simulink library "MERMASS11MSEREF"  (R2020b)
settings: Solver=ode45  StartTime=0.0  StopTime=10.0  RelTol=1e-3  EnableMultiTasking=on
settings Model: Creator=vda2sh  LastModifiedBy=CAV2OFO
settings DataIOCC: LimitDataPoints=on  SaveFormat=Array  ReturnWorkspaceOutputs=off
settings OptimizationCC: LifeSpan=inf
settings DebuggingCC: SolverPrmCheckMsg=warning  SFUnexpectedBacktrackingDiag=warning  SFNoUnconditionalDefaultTransitionDiag=warning  SFExecutionAtInitializationDiag=none  ArithmeticOperatorsInVariantConditions=warning
settings HardwareCC: ProdBitPerPointer=32  ProdBitPerSizeT=32  ProdBitPerPtrDiffT=32  ProdLargestAtomicFloat=None  ProdIntDivRoundTo=Undefined  ProdEndianess=Unspecified  ProdWordSize=32  ProdHWDeviceType=32-bit Generic
settings ModelReferenceCC: PropagateSignalLabelsOutOfModel=off
settings SFSimCC: SimUseLocalCustomCode=off  CustomCodeUndefinedFunction=UseInterfaceOnly
settings RTWCC: RTWUseLocalCustomCode=off
settings CodeAppCC: StateflowObjectComments=on
settings GRTTargetCC: TargetLangStandard=C89/C90 (ANSI)
settings ConfigComp: CovMetricSettings=dw  CovSaveCumulativeToWorkspaceVar=on  CovSaveSingleToWorkspaceVar=on  CovExternalEMLEnable=off  CovSFcnEnable=off

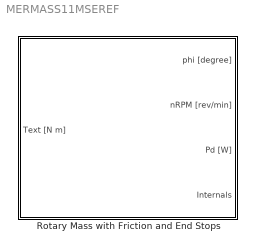
== system MERMASS11MSEREF ==
  Rotary Mass with Friction and End Stops : Subsystem  Tag=MERMASS11MSEREF  mask(MERMASS11MSEREF){J=1.625e-5, dvisc=0.001, frictionmode=no friction, epsn=0.001, tauinv=1000, TStick=1, TCoulomb=0.9, nStri=0.01, endstopmode=no end stop, phimin=-1e6, phimax=1e6, cstop=1e6, kimpact=0.5, phiinit=0, nRPMinit=0}
      mask prompts: J "Inertia [kg m2]"; dvisc "Viscous damping [N m/(rev/min)]"; frictionmode "Friction mode"; epsn "Numerical parameter for friction treatment [rev/min]"; tauinv "Inverse of time constant at stiction (variable step solvers only) [1/s]"; TStick "Torque at stick friction [N m]"; TCoulomb "Torque at Coulomb friction [N m]"; nStri "Stribeck rotational speed [rev/min]"; endstopmode "End stop mode"; phimin "Lower angular displacement limit [°]"; phimax "Upper angular displacement limit [°]"; cstop "Spring coefficient at displacement limit [N m/°]"; kimpact "Coefficient of restitution [-]"; phiinit "Initial displacement [°]"; nRPMinit "Initial rotational speed [rev/min]"
      mask help:
      | MERMASS11MSEREF - Rotary Mass with Friction and End Stops
      |
      | This is a model of a mass in rotary motion with friction effects and inertia. The displacement of the mass may be limited by lower and upper values. One detailed model of friction is implemented, as well as one model for the phenomenon of end stop.
      settings: AttributesFormatString=<%<Tag>>
      mask Help: eval('show_docs_mseref_mechanics(''MERMASS11MSEREF'')')
      mask TypeOptions frictionmode: no friction | stribeck + slip/Coulomb friction
      mask Callback frictionmode:
      | MCBVP__.endstopmode = get_param(gcb,'endstopmode');
      | 
      | MCBVP__.frictionmode = get_param(gcb,'frictionmode');
      | 
      | 		MCBVP__.enables = {};
      | 		MCBVP__.visibilities = {};
      | 
      | 				MCBVP__.enables{end + 1} = 'on';
      | 				MCBVP__.visibilities{end + 1} = 'on';
      | 
      | 				MCBVP__.enables{end + 1} = 'on';
      | 				MCBVP__.visibilities{end + 1} = 'on';
      | 
      | 				MCBVP__.enables{end + 1} = 'on';
      | 				MCBVP__.visibilities{end + 1} = 'on';
      | 
      | 				if strcmp(MCBVP__.frictionmode,'stribeck + slip/Coulomb friction')
      | 					MCBVP__.enables{end + 1} = 'on';
      | 					MCBVP__.visibilities{end + 1} = 'on';
      | 				else
      | 					MCBVP__.enables{end + 1} = 'off';
      | 					MCBVP__.visibilities{end + 1} = 'off';
      | 				end
      | 
      | 				if strcmp(MCBVP__.frictionmode,'stribeck + slip/Coulomb friction')
      | 					MCBVP__.enables{end + 1} = 'on';
      | 					MCBVP__.visibilities{end + 1} = 'on';
      | 				else
      | 					MCBVP__.enables{end + 1} = 'off';
      | 					MCBVP__.visibilities{end + 1} = 'off';
      | 				end
      | 
      | 				if strcmp(MCBVP__.frictionmode,'stribeck + slip/Coulomb friction')
      | 					MCBVP__.enables{end + 1} = 'on';
      | 					MCBVP__.visibilities{end + 1} = 'on';
      | 				else
      | 					MCBVP__.enables{end + 1} = 'off';
      | 					MCBVP__.visibilities{end + 1} = 'off';
      | 				end
      | 
      | 				if strcmp(MCBVP__.frictionmode,'stribeck + slip/Coulomb friction')
      | 					MCBVP__.enables{end + 1} = 'on';
      | 					MCBVP__.visibilities{end + 1} = 'on';
      | 				else
      | 					MCBVP__.enables{end + 1} = 'off';
      | 					MCBVP__.visibilities{end + 1} = 'off';
      | 				end
      | 
      | 				if strcmp(MCBVP__.frictionmode,'stribeck + slip/Coulomb friction')
      | 					MCBVP__.enables{end + 1} = 'on';
      | 					MCBVP__.visibilities{end + 1} = 'on';
      | 				else
      | 					MCBVP__.enables{end + 1} = 'off';
      | 					MCBVP__.visibilities{end + 1} = 'off';
      | 				end
      | 
      | 				MCBVP__.enables{end + 1} = 'on';
      | 				MCBVP__.visibilities{end + 1} = 'on';
      | 
      | 				if ~(strcmp(MCBVP__.endstopmode,'no end stop'))
      | 					MCBVP__.enables{end + 1} = 'on';
      | 					MCBVP__.visibilities{end + 1} = 'on';
      | 				else
      | 					MCBVP__.enables{end + 1} = 'off';
      | 					MCBVP__.visibilities{end + 1} = 'off';
      | 				end
      | 
      | 				if ~(strcmp(MCBVP__.endstopmode,'no end stop'))
      | 					MCBVP__.enables{end + 1} = 'on';
      | 					MCBVP__.visibilities{end + 1} = 'on';
      | 				else
      | 					MCBVP__.enables{end + 1} = 'off';
      | 					MCBVP__.visibilities{end + 1} = 'off';
      | 				end
      | 
      | 				if ~(strcmp(MCBVP__.endstopmode,'no end stop'))
      | 					MCBVP__.enables{end + 1} = 'on';
      | 					MCBVP__.visibilities{end + 1} = 'on';
      | 				else
      | 					MCBVP__.enables{end + 1} = 'off';
      | 					MCBVP__.visibilities{end + 1} = 'off';
      | 				end
      | 
      | 				if ~(strcmp(MCBVP__.endstopmode,'no end stop'))
      | 					MCBVP__.enables{end + 1} = 'on';
      | 					MCBVP__.visibilities{end + 1} = 'on';
      | 				else
      | 					MCBVP__.enables{end + 1} = 'off';
      | 					MCBVP__.visibilities{end + 1} = 'off';
      | 				end
      | 
      | 				MCBVP__.enables{end + 1} = 'on';
      | 				MCBVP__.visibilities{end + 1} = 'on';
      | 
      | 				MCBVP__.enables{end + 1} = 'on';
      | 				MCBVP__.visibilities{end + 1} = 'on';
      | 
      | 		set_param(gcb, 'MaskEnables', MCBVP__.enables);
      | 		set_param(gcb, 'MaskVisibilities', MCBVP__.visibilities);
      | 		clear MCBVP__;
      mask TypeOptions endstopmode: no end stop | elastic
      mask Callback endstopmode:
      | MCBVP__.endstopmode = get_param(gcb,'endstopmode');
      | 
      | MCBVP__.frictionmode = get_param(gcb,'frictionmode');
      | 
      | 		MCBVP__.enables = {};
      | 		MCBVP__.visibilities = {};
      | 
      | 				MCBVP__.enables{end + 1} = 'on';
      | 				MCBVP__.visibilities{end + 1} = 'on';
      | 
      | 				MCBVP__.enables{end + 1} = 'on';
      | 				MCBVP__.visibilities{end + 1} = 'on';
      | 
      | 				MCBVP__.enables{end + 1} = 'on';
      | 				MCBVP__.visibilities{end + 1} = 'on';
      | 
      | 				if strcmp(MCBVP__.frictionmode,'stribeck + slip/Coulomb friction')
      | 					MCBVP__.enables{end + 1} = 'on';
      | 					MCBVP__.visibilities{end + 1} = 'on';
      | 				else
      | 					MCBVP__.enables{end + 1} = 'off';
      | 					MCBVP__.visibilities{end + 1} = 'off';
      | 				end
      | 
      | 				if strcmp(MCBVP__.frictionmode,'stribeck + slip/Coulomb friction')
      | 					MCBVP__.enables{end + 1} = 'on';
      | 					MCBVP__.visibilities{end + 1} = 'on';
      | 				else
      | 					MCBVP__.enables{end + 1} = 'off';
      | 					MCBVP__.visibilities{end + 1} = 'off';
      | 				end
      | 
      | 				if strcmp(MCBVP__.frictionmode,'stribeck + slip/Coulomb friction')
      | 					MCBVP__.enables{end + 1} = 'on';
      | 					MCBVP__.visibilities{end + 1} = 'on';
      | 				else
      | 					MCBVP__.enables{end + 1} = 'off';
      | 					MCBVP__.visibilities{end + 1} = 'off';
      | 				end
      | 
      | 				if strcmp(MCBVP__.frictionmode,'stribeck + slip/Coulomb friction')
      | 					MCBVP__.enables{end + 1} = 'on';
      | 					MCBVP__.visibilities{end + 1} = 'on';
      | 				else
      | 					MCBVP__.enables{end + 1} = 'off';
      | 					MCBVP__.visibilities{end + 1} = 'off';
      | 				end
      | 
      | 				if strcmp(MCBVP__.frictionmode,'stribeck + slip/Coulomb friction')
      | 					MCBVP__.enables{end + 1} = 'on';
      | 					MCBVP__.visibilities{end + 1} = 'on';
      | 				else
      | 					MCBVP__.enables{end + 1} = 'off';
      | 					MCBVP__.visibilities{end + 1} = 'off';
      | 				end
      | 
      | 				MCBVP__.enables{end + 1} = 'on';
      | 				MCBVP__.visibilities{end + 1} = 'on';
      | 
      | 				if ~(strcmp(MCBVP__.endstopmode,'no end stop'))
      | 					MCBVP__.enables{end + 1} = 'on';
      | 					MCBVP__.visibilities{end + 1} = 'on';
      | 				else
      | 					MCBVP__.enables{end + 1} = 'off';
      | 					MCBVP__.visibilities{end + 1} = 'off';
      | 				end
      | 
      | 				if ~(strcmp(MCBVP__.endstopmode,'no end stop'))
      | 					MCBVP__.enables{end + 1} = 'on';
      | 					MCBVP__.visibilities{end + 1} = 'on';
      | 				else
      | 					MCBVP__.enables{end + 1} = 'off';
      | 					MCBVP__.visibilities{end + 1} = 'off';
      | 				end
      | 
      | 				if ~(strcmp(MCBVP__.endstopmode,'no end stop'))
      | 					MCBVP__.enables{end + 1} = 'on';
      | 					MCBVP__.visibilities{end + 1} = 'on';
      | 				else
      | 					MCBVP__.enables{end + 1} = 'off';
      | 					MCBVP__.visibilities{end + 1} = 'off';
      | 				end
      | 
      | 				if ~(strcmp(MCBVP__.endstopmode,'no end stop'))
      | 					MCBVP__.enables{end + 1} = 'on';
      | 					MCBVP__.visibilities{end + 1} = 'on';
      | 				else
      | 					MCBVP__.enables{end + 1} = 'off';
      | 					MCBVP__.visibilities{end + 1} = 'off';
      | 				end
      | 
      | 				MCBVP__.enables{end + 1} = 'on';
      | 				MCBVP__.visibilities{end + 1} = 'on';
      | 
      | 				MCBVP__.enables{end + 1} = 'on';
      | 				MCBVP__.visibilities{end + 1} = 'on';
      | 
      | 		set_param(gcb, 'MaskEnables', MCBVP__.enables);
      | 		set_param(gcb, 'MaskVisibilities', MCBVP__.visibilities);
      | 		clear MCBVP__;
      mask DialogControl ParameterTabVar0 Prompt: Parameters
      mask DialogControl ParameterTabVar01 Prompt: Initial values
      mask Display:
      | image(imread('MERMASS11MSEREF.png'),[0.23, 0.005, 0.58, 0.58])
      | port_label('input',1,'Text [N m]')
      | port_label('output',1,'phi [degree]')
      | port_label('output',2,'nRPM [rev/min]')
      | port_label('output',3,'Pd [W]')
      | port_label('output',4,'Internals')

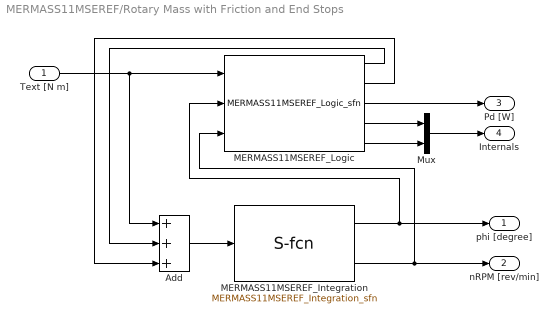
== system MERMASS11MSEREF/Rotary Mass with Friction and End Stops ==
  Text [N m] : Inport
  Add : Sum  Inputs=+++
  MERMASS11MSEREF_Integration : S-Function  FunctionName=MERMASS11MSEREF_Integration_sfn  Parameters=phiinit, nRPMinit, J  SFunctionDeploymentMode=off  EnableBusSupport=off  mask{phinit=phiinit, nRPMinit=nRPMinit, J=J}
      mask prompts: phinit "Initial Angular displacement [deg]"; nRPMinit "Initial Rotational speed [rev/min]"; J "Inertia [kgm2]"
      mask Display:
      | port_label('input',1,'Tsum')
      | port_label('output',1,'phiOut')
      | port_label('output',2,'nRPM')
  MERMASS11MSEREF_Logic : S-Function  FunctionName=MERMASS11MSEREF_Logic_sfn  Parameters=phiinit, J, dvisc, frictionmode, epsn, tauinv, TStick, TCoulomb, nStri, endstopmode, phimin, phimax, cstop, kimpact  SFunctionDeploymentMode=off  EnableBusSupport=off  mask{phiinit=phiinit, J=J, dvisc=dvisc, frictionmode=frictionmode, epsn=epsn, tauinv=tauinv, TStick=TStick, TCoulomb=TCoulomb, nStri=nStri, endstopmode=endstopmode, phimin=phimin, phimax=phimax, cstop=cstop, kimpact=kimpact}
      mask prompts: phiinit "Initial angular displacement [deg]"; J "Inertia [kg m^2]"; dvisc "Viscous damping [Nm/(rev/min)]"; frictionmode "Friction mode"; epsn "Numerical parameter for friction treatment [rev/min]"; tauinv "Inverse of time constant for numerical damping at stiction [1/s]"; TStick "Torque at stick friction [Nm]"; TCoulomb "Torque at Coulomb friction [Nm]"; nStri "Stribeck rotational speed [rev/min]"; endstopmode "End stop mode"; phimin "Lower angular displacement limit [deg]"; phimax "Upper angular displacement limit [deg]"; cstop "Spring coefficient at displacement limit [Nm/deg]"; kimpact "Coefficient of restitution [-]"
      mask Display:
      | port_label('input',1,'Text')
      | port_label('input',2,'phi')
      | port_label('input',3,'nRPM')
      | port_label('output',1,'Tfr')
      | port_label('output',2,'Tstop')
      | port_label('output',3,'Pd')
      | port_label('output',4,'DSfrOut')
      | port_label('output',5,'DSendstopOut')
  Mux : Mux  Inputs=2
  phi [degree] : Outport
  nRPM [rev/min] : Outport  Port=2
  Pd [W] : Outport  Port=3
  Internals : Outport  Port=4
  wires:
  Mux/1 -> Internals/1
  MERMASS11MSEREF_Logic/5 -> Mux/2
  MERMASS11MSEREF_Logic/4 -> Mux/1
  MERMASS11MSEREF_Logic/3 -> Pd [W]/1
  MERMASS11MSEREF_Logic/2 -> Add/3
  MERMASS11MSEREF_Logic/1 -> Add/2
  Text [N m]/1 -> Add/1, MERMASS11MSEREF_Logic/1
  MERMASS11MSEREF_Integration/2 -> MERMASS11MSEREF_Logic/3, nRPM [rev/min]/1
  MERMASS11MSEREF_Integration/1 -> MERMASS11MSEREF_Logic/2, phi [degree]/1
  Add/1 -> MERMASS11MSEREF_Integration/1
